simulink model "test"  (R2025b)
settings: Solver=VariableStepAuto  StartTime=0.0  StopTime=10.0  RelTol=1e-3
values from neighbouring files (symbols this model uses):
  A_1 = [zeros(2) eye(2) ... (first row only)    [model.m]
  B_1 = [0;0 ... (first row only)    [model.m]
  gamma = 0.999    [model.m]
  H_barre = K_t(5)    [model.m]
  K_int = K_t(1:4)    [model.m]
  K_PWM = 8.087    [model.m]
  Psi0 = deg2rad(8)    [model.m]
  s1 = ss(A_1, B_1, eye(4), zeros(4,1))    [model.m]
  Ts = 0.004    [model.m]
undefined symbols (not defined in the file or in its folder): DiscIntNeverNeededParam
libraries: simulink x1
settings Model: Creator=carol  LastModifiedBy=carol

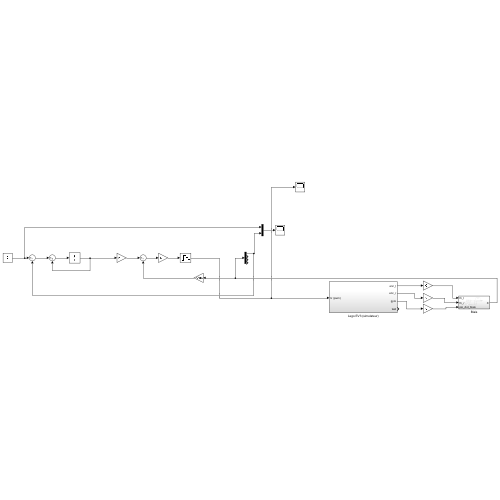
[thumbnail: Simulink's stored preview of the top-level diagram]
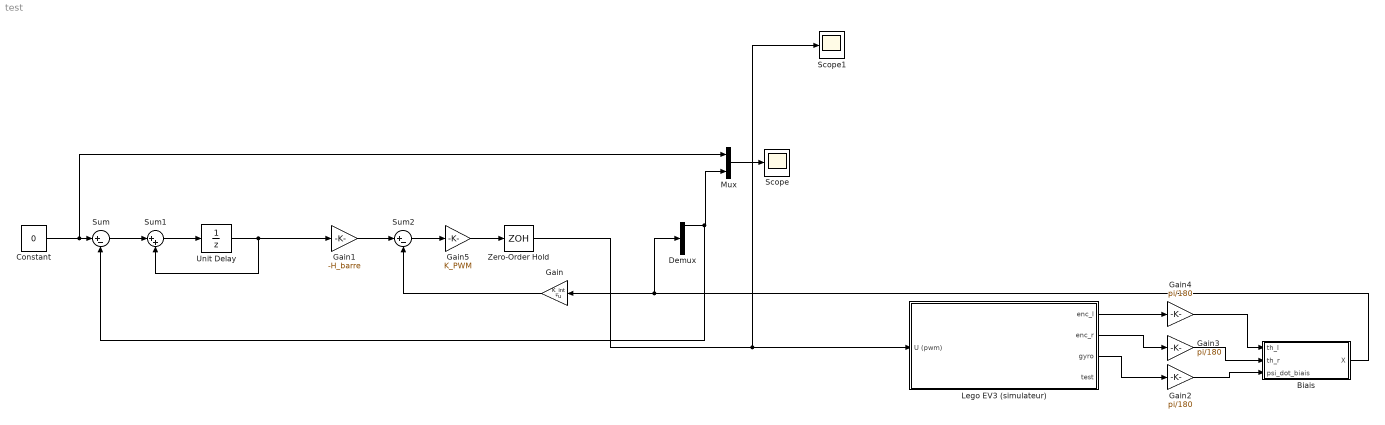
== system test ==
  Biais : Subsystem
  Constant : Constant  Value=0
  Demux : Demux
  Gain : Gain  Gain=K_int  Multiplication=Matrix(K*u) (u vector)
  Gain1 : Gain  Gain=-H_barre
  Gain2 : Gain  Gain=pi/180
  Gain3 : Gain  Gain=pi/180
  Gain4 : Gain  Gain=pi/180
  Gain5 : Gain  Gain=K_PWM
  Lego EV3 (simulateur) : Subsystem
  Mux : Mux  Inputs=2
  Scope : Scope
      settings: ActiveDisplayYMinimum=-7.2146783078767182E+28  ActiveDisplayYMaximum=8.0163092309741288E+27
  Scope1 : Scope
  Sum : Sum  Inputs=|+-
  Sum1 : Sum  Inputs=|++
  Sum2 : Sum  Inputs=|+-
  Unit Delay : UnitDelay  SampleTime=-1  HasFrameUpgradeWarning=on
  Zero-Order Hold : ZeroOrderHold  SampleTime=Ts
  wires:
  Biais/1(X) -> Demux/1, Gain/1
  Sum2/1 -> Gain5/1
  Gain/1 -> Sum2/2
  Zero-Order Hold/1 -> Scope1/1, Lego EV3 (simulateur)/1(U (pwm))
  Gain1/1 -> Sum2/1
  Demux/1 -> Mux/2, Sum/2
  Mux/1 -> Scope/1
  Constant/1 -> Mux/1, Sum/1
  Sum1/1 -> Unit Delay/1
  Unit Delay/1 -> Sum1/2, Gain1/1
  Sum/1 -> Sum1/1
  Gain3/1 -> Biais/2(th_r)
  Lego EV3 (simulateur)/2(enc_r) -> Gain3/1
  Lego EV3 (simulateur)/1(enc_l) -> Gain4/1
  Lego EV3 (simulateur)/3(gyro) -> Gain2/1
  Gain4/1 -> Biais/1(th_l)
  Gain5/1 -> Zero-Order Hold/1
  Gain2/1 -> Biais/3(psi_dot_biais)

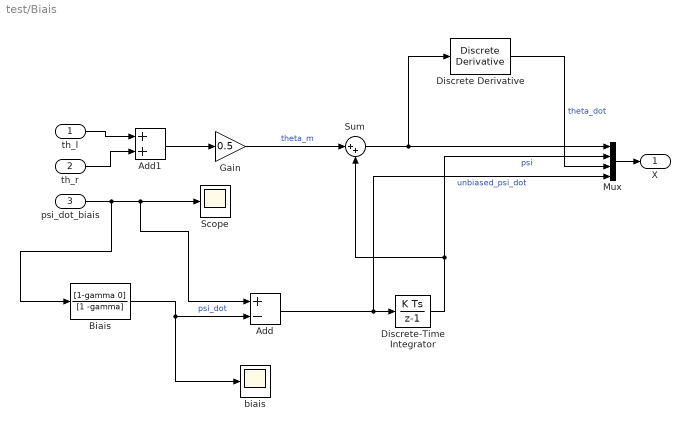
== system test/Biais ==
  th_l : Inport
  th_r : Inport  Port=2
  psi_dot_biais : Inport  Port=3
  Add : Sum  Inputs=+-
  Add1 : Sum
  Biais : DiscreteTransferFcn  Numerator=[1-gamma 0]  Denominator=[1 -gamma]
  Discrete Derivative : simulink/Quick Insert/Discrete/Discrete Derivative  gainval=1.0  ICPrevScaledInput=0.0  OutMin=[]  OutMax=[]  OutDataType=fixdt(1, 16)  OutScaling=2^-10  DoSatur=off
  Discrete-Time Integrator : DiscreteIntegrator  SampleTime=Ts  ICPrevOutput=DiscIntNeverNeededParam  ICPrevScaledInput=DiscIntNeverNeededParam
  Gain : Gain  Gain=0.5
  Mux : Mux
  Scope : Scope
      settings: ActiveDisplayYMinimum=-1  ActiveDisplayYMaximum=1  DataLoggingVariableName=ScopeData13
  Sum : Sum  Inputs=|++
  biais : Scope
      settings: ActiveDisplayYMinimum=-0.1164059395354744  ActiveDisplayYMaximum=0.0646369691442869  DataLoggingVariableName=ScopeData12
  X : Outport
  wires:
  th_l/1 -> Add1/1
  th_r/1 -> Add1/2
  Add1/1 -> Gain/1
  Mux/1 -> X/1
  Discrete Derivative/1 -> Mux/3  "theta_dot"
  Discrete-Time Integrator/1 -> Sum/2, Mux/2  "psi"
  psi_dot_biais/1 -> Biais/1, Add/1, Scope/1
  Biais/1 -> Add/2, biais/1  "psi_dot"
  Add/1 -> Mux/4, Discrete-Time Integrator/1  "unbiased_psi_dot"
  Gain/1 -> Sum/1  "theta_m"
  Sum/1 -> Mux/1, Discrete Derivative/1

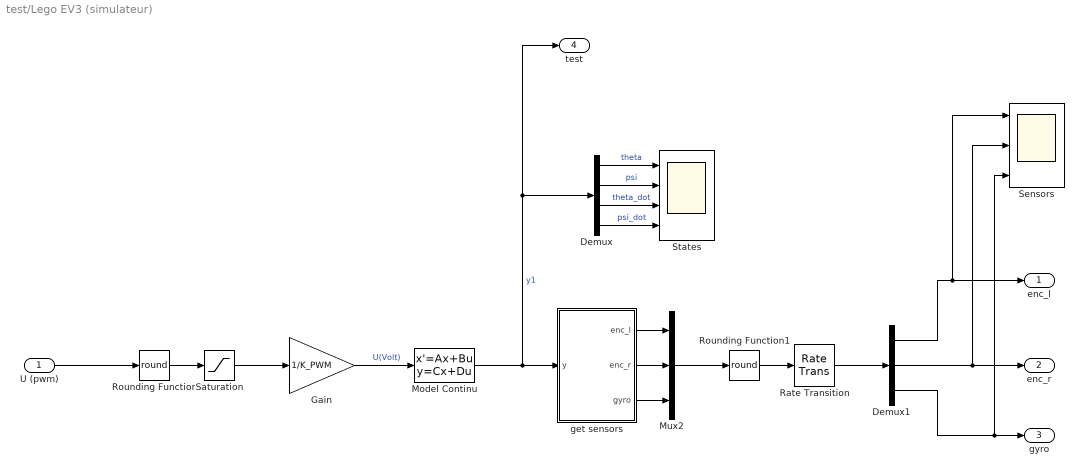
== system test/Lego EV3 (simulateur) ==
  U (pwm) : Inport
  Demux : Demux
  Demux1 : Demux  Outputs=3
  Gain : Gain  Gain=1/K_PWM
  Model Continu : StateSpace  A=A_1  B=B_1  C=eye(4)  D=s1.D  InitialCondition=[0 Psi0 0 0]
  Mux2 : Mux  Inputs=3
  Rate Transition : RateTransition  OutPortSampleTime=Ts
  Rounding Function : Rounding  Operator=round
  Rounding Function1 : Rounding  Operator=round
  Saturation : Saturate  UpperLimit=100  LowerLimit=-100
  Sensors : Scope  NumInputPorts=3
      settings: ActiveDisplayYMinimum=-115  ActiveDisplayYMaximum=265
  States : Scope  NumInputPorts=4
      settings: ActiveDisplayYMinimum=-18.762173178074935  ActiveDisplayYMaximum=8.1937673053565856  DataLoggingVariableName=ScopeData2
  get sensors : MATLAB Function  TreatAsAtomicUnit=on
  enc_l : Outport
  enc_r : Outport  Port=2
  gyro : Outport  Port=3
  test : Outport  Port=4
  wires:
  Model Continu/1 -> test/1, Demux/1, get sensors/1(y)  "y1"
  Gain/1 -> Model Continu/1  "U(Volt)"
  Saturation/1 -> Gain/1
  U (pwm)/1 -> Rounding Function/1
  get sensors/3(gyro) -> Mux2/3
  Demux/4 -> States/4  "psi_dot"
  Rounding Function1/1 -> Rate Transition/1
  Demux/2 -> States/2  "psi"
  Demux/3 -> States/3  "theta_dot"
  Demux/1 -> States/1  "theta"
  get sensors/1(enc_l) -> Mux2/1
  get sensors/2(enc_r) -> Mux2/2
  Rounding Function/1 -> Saturation/1
  Mux2/1 -> Rounding Function1/1
  Rate Transition/1 -> Demux1/1
  Demux1/1 -> Sensors/1, enc_l/1
  Demux1/2 -> Sensors/2, enc_r/1
  Demux1/3 -> Sensors/3, gyro/1

== matlab function test/Lego EV3 (simulateur)/get sensors ==
  data: enc_l output; enc_r output; y input; gyro output; R parameter
function [enc_l, enc_r, gyro] = sensors(y, R)
enc_l = rad2deg(y(1) - y(2));
enc_r = rad2deg(y(1) - y(2));
gyro  = rad2deg(y(4));
